simulink model "final11"  (R2015b)
settings: Solver=FixedStepAuto  StartTime=0.0  StopTime=0.002  FixedStep=1e-10  RelTol=1e-3
libraries: dsparch4 x2, commsynccomp2 x2, dspxfrm3 x1, rfmathmodels1 x1, rfprivate1 x1
settings Model: Creator=dimple  LastModifiedBy=dimple

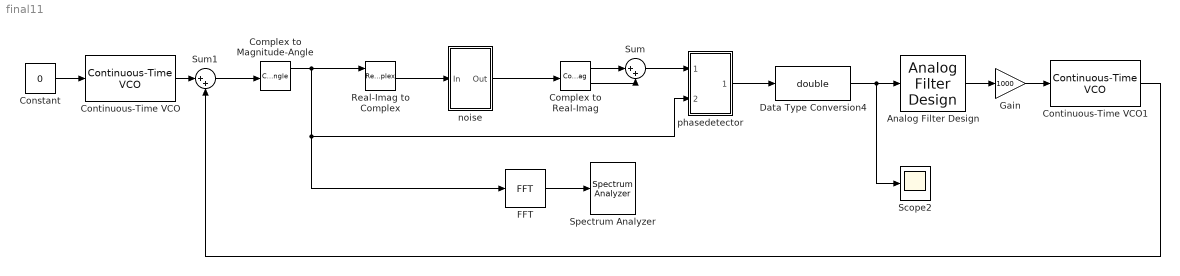
== system final11 ==
  Analog Filter Design : dsparch4/Analog Filter Design  method=Butterworth  filttype=Lowpass  N=8  Wlo=1e2  Whi=80  Rp=2  Rs=40
  Complex to Magnitude-Angle : ComplexToMagnitudeAngle
  Complex to Real-Imag : ComplexToRealImag
  Constant : Constant  Value=0
  Continuous-Time VCO : commsynccomp2/Continuous-Time VCO  Ac=10  Fc=1e9  Kc=1e8  Ph=0
  Continuous-Time VCO1 : commsynccomp2/Continuous-Time VCO  Ac=10  Fc=1.25e9  Kc=1e8  Ph=0
  Data Type Conversion4 : DataTypeConversion  OutDataTypeStr=double
  FFT : dspxfrm3/FFT  FFTImplementation=Auto  CompMethod=Table lookup  TableOpt=NEW  TableOptActive=Speed  BitRevOrder=off  Normalize=off  InheritFFTLength=on  FFTLength=64  WrapInput=on  roundingMode=Floor  overflowMode=off  firstCoeffDataTypeStr=Inherit: Same word length as input  firstCoeffLastDataTypeStr=Inherit: Same word length as input  outputMin=[]  outputMax=[]
  Gain : Gain  Gain=1000
  Real-Imag to Complex : RealImagToComplex
  Scope2 : Scope
  Spectrum Analyzer : SpectrumAnalyzer
  Sum : Sum  Inputs=|++
  Sum1 : Sum  Inputs=|++
  "noise " : Subsystem
  "phasedetector " : Subsystem
  wires:
  Continuous-Time VCO/1 -> Sum1/1
  Real-Imag to Complex/1 -> "noise "/1(In)
  Constant/1 -> Continuous-Time VCO/1
  "noise "/1(Out) -> Complex to Real-Imag/1
  Sum/1 -> "phasedetector "/1(In1)
  Data Type Conversion4/1 -> Scope2/1, Analog Filter Design/1
  Continuous-Time VCO1/1 -> Sum1/2
  "phasedetector "/1(Out1) -> Data Type Conversion4/1
  FFT/1 -> Spectrum Analyzer/1
  Sum1/1 -> Complex to Magnitude-Angle/1
  Complex to Magnitude-Angle/1 -> FFT/1, "phasedetector "/2(In2), Real-Imag to Complex/1
  Gain/1 -> Continuous-Time VCO1/1
  Analog Filter Design/1 -> Gain/1
  Complex to Real-Imag/1 -> Sum/1
  Complex to Real-Imag/2 -> Sum/2

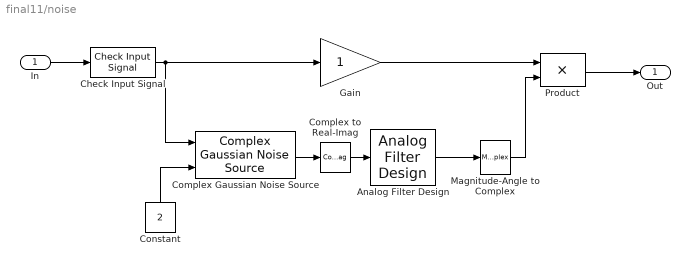
== system final11/noise  ==
  In : Inport
  Analog Filter Design : dsparch4/Analog Filter Design  method=Butterworth  filttype=Lowpass  N=5  Wlo=1e7  Whi=80  Rp=2  Rs=40
  Check Input Signal : rfmathmodels1/Mixer/Check Input Signal  SystemSampleTime=-1
  Complex Gaussian Noise Source : rfprivate1/Complex Gaussian Noise Source  myseed=2137
  Complex to Real-Imag : ComplexToRealImag  Output=Real
  Constant : Constant  Value=2
  Gain : Gain  SaturateOnIntegerOverflow=on  OutDataTypeStr=Inherit: Same as input  ParamDataTypeStr=Inherit: Same as input
  Magnitude-Angle to Complex : MagnitudeAngleToComplex  Input=Angle  ConstantPart=1
  Product : Product  SaturateOnIntegerOverflow=on  InputSameDT=on  OutDataTypeStr=Inherit: Same as first input
  Out : Outport
  wires:
  Constant/1 -> Complex Gaussian Noise Source/2
  Complex Gaussian Noise Source/1 -> Complex to Real-Imag/1
  Gain/1 -> Product/1
  Check Input Signal/1 -> Complex Gaussian Noise Source/1, Gain/1
  In/1 -> Check Input Signal/1
  Product/1 -> Out/1
  Complex to Real-Imag/1 -> Analog Filter Design/1
  Magnitude-Angle to Complex/1 -> Product/2
  Analog Filter Design/1 -> Magnitude-Angle to Complex/1

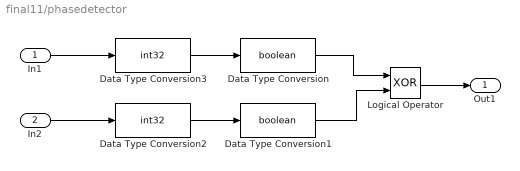
== system final11/phasedetector  ==
  In1 : Inport
  In2 : Inport  Port=2
  Data Type Conversion : DataTypeConversion  OutDataTypeStr=boolean
  Data Type Conversion1 : DataTypeConversion  OutDataTypeStr=boolean
  Data Type Conversion2 : DataTypeConversion  OutDataTypeStr=int32
  Data Type Conversion3 : DataTypeConversion  OutDataTypeStr=int32
  Logical Operator : Logic  Operator=XOR  AllPortsSameDT=off  OutDataTypeStr=boolean
  Out1 : Outport
  wires:
  Data Type Conversion3/1 -> Data Type Conversion/1
  Logical Operator/1 -> Out1/1
  Data Type Conversion/1 -> Logical Operator/1
  Data Type Conversion1/1 -> Logical Operator/2
  In1/1 -> Data Type Conversion3/1
  Data Type Conversion2/1 -> Data Type Conversion1/1
  In2/1 -> Data Type Conversion2/1
